simulink model "ChargerSystem"  (R2018a)
settings: Solver=FixedStepDiscrete  StartTime=0.0  StopTime=inf  RelTol=1e-3
libraries: arduinolib x8, simulink x1
settings Model: SimulationMode=external  ExtModeTrigDuration=2  Creator=fabricek  LastModifiedBy=fabricek
settings SolverCC: AutoInsertRateTranBlk=on
settings DataIOCC: SignalLogging=off
settings OptimizationCC: EnhancedBackFolding=on  PassReuseOutputArgsThreshold=0  MaxStackSize=64  OptimizeBlockOrder=speed  DifferentSizesBufferReuse=on  OptimizationCustomize=off
settings DebuggingCC: ParameterTunabilityLossMsg=error
settings HardwareCC: ProdBitPerInt=16  ProdBitPerPointer=16  ProdBitPerSizeT=16  ProdBitPerPtrDiffT=16  ProdLargestAtomicFloat=None  ProdWordSize=8  ProdHWDeviceType=Atmel->AVR  UseEmbeddedCoderFeatures=off  UseSimulinkCoderFeatures=off
settings SFSimCC: MATLABDynamicMemAlloc=off
settings RTWCC: SystemTargetFile=ert.tlc  HardwareBoard=Arduino Uno  TLCOptions=-aInlineSetEventsForThisBaseRateFcn=TLC_FALSE -aSuppressMultiTaskScheduler=TLC_FALSE -aRateBasedStepFcn=1  TemplateMakefile=ert_default_tmf  GenerateReport=on  Toolchain=Arduino AVR  BuildConfiguration=Faster Runs  LaunchReport=on
settings CodeAppCC: ForceParamTrailComments=on  OperatorAnnotations=on
settings ERTTargetCC: ERTCustomFileBanners=off  SupportContinuousTime=on  SupportNonInlinedSFcns=on  RemoveResetFunc=off  SupportVariableSizeSignals=on  ModelStepFunctionPrototypeControlCompliant=off

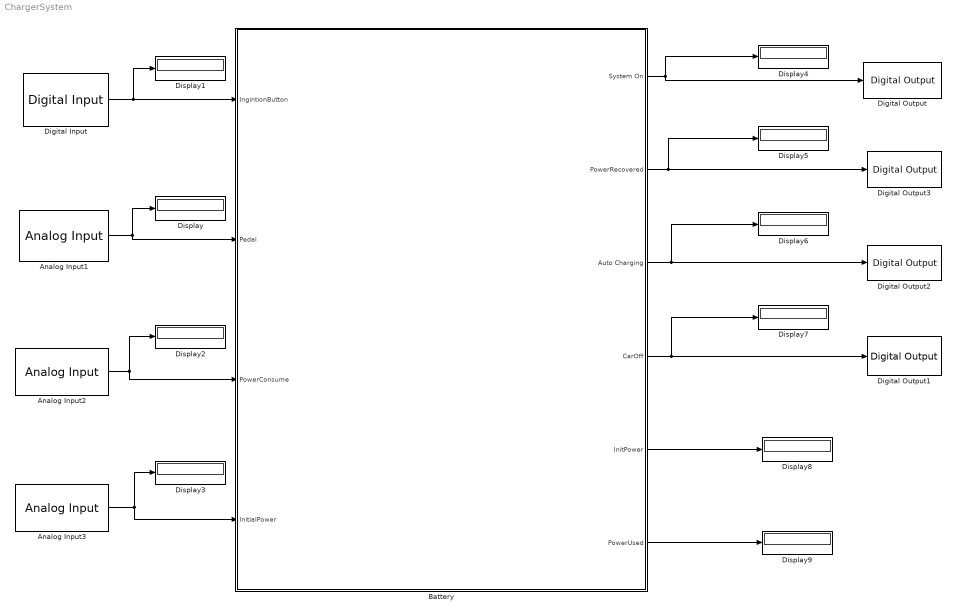
== system ChargerSystem ==
  Analog Input1 : arduinolib/Analog Input  pinNumber=2  ReadResultsOnly=off  ConversionTriggerSource=Software  ExternalTriggerType=uint32(0)  OutputDataType=uint16  EnableConversionCompleteNotify=off  EnableOuputStatus=off  SampleTime=1  blockPlatform=arduino
  Analog Input2 : arduinolib/Analog Input  pinNumber=1  ReadResultsOnly=off  ConversionTriggerSource=Software  ExternalTriggerType=uint32(0)  OutputDataType=uint16  EnableConversionCompleteNotify=off  EnableOuputStatus=off  SampleTime=1  blockPlatform=arduino
  Analog Input3 : arduinolib/Analog Input  pinNumber=0  ReadResultsOnly=off  ConversionTriggerSource=Software  ExternalTriggerType=uint32(0)  OutputDataType=uint16  EnableConversionCompleteNotify=off  EnableOuputStatus=off  SampleTime=1  blockPlatform=arduino
  Battery : Subsystem
  Digital Input : arduinolib/Digital Input  pinNumber=13  sampleTime=0.1  blockPlatform=arduino
      settings: SourceProductName=Simulink Support Package for Arduino Hardware
  Digital Output : arduinolib/Digital Output  pinNumber=9  blockPlatform=arduino
  Digital Output1 : arduinolib/Digital Output  pinNumber=2  blockPlatform=arduino
  Digital Output2 : arduinolib/Digital Output  pinNumber=4  blockPlatform=arduino
  Digital Output3 : arduinolib/Digital Output  pinNumber=7  blockPlatform=arduino
  Display{,1..9} (10 alike) : Display
  wires:
  Battery/6(PowerUsed) -> Display9/1
  Analog Input2/1 -> Battery/3(PowerConsume), Display2/1
  Battery/2(PowerRecovered) -> Display5/1, Digital Output3/1
  Analog Input3/1 -> Battery/4(InitialPower), Display3/1
  Battery/5(InitPower) -> Display8/1
  Battery/1(System On) -> Digital Output/1, Display4/1
  Battery/3(Auto Charging) -> Display6/1, Digital Output2/1
  Battery/4(CarOff) -> Display7/1, Digital Output1/1
  Analog Input1/1 -> Battery/2(Pedal), Display/1
  Digital Input/1 -> Battery/1(IngintionButton), Display1/1

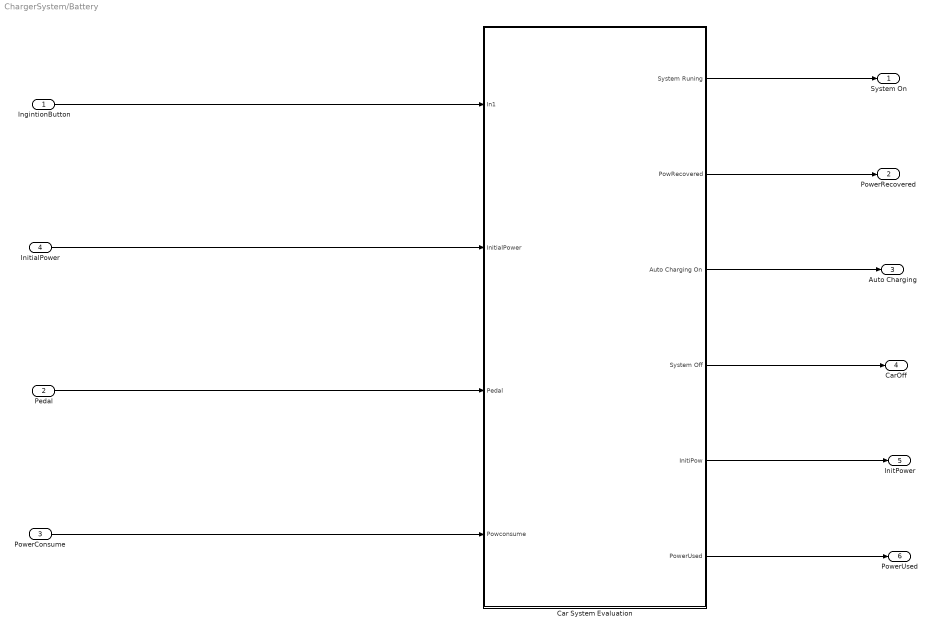
== system ChargerSystem/Battery ==
  IngintionButton : Inport
  Pedal : Inport  Port=2
  PowerConsume : Inport  Port=3
  InitialPower : Inport  Port=4
  Car System Evaluation : Subsystem
  System On : Outport
  PowerRecovered : Outport  Port=2
  Auto Charging : Outport  Port=3
  CarOff : Outport  Port=4
  InitPower : Outport  Port=5
  PowerUsed : Outport  Port=6
  wires:
  IngintionButton/1 -> Car System Evaluation/1(In1)
  Car System Evaluation/4(System Off) -> CarOff/1
  Car System Evaluation/1(System Runing) -> System On/1
  Car System Evaluation/2(PowRecovered) -> PowerRecovered/1
  Car System Evaluation/3(Auto Charging On) -> Auto Charging/1
  Pedal/1 -> Car System Evaluation/3(Pedal)
  PowerConsume/1 -> Car System Evaluation/4(Powconsume)
  InitialPower/1 -> Car System Evaluation/2(InitialPower)
  Car System Evaluation/5(InitiPow) -> InitPower/1
  Car System Evaluation/6(PowerUsed) -> PowerUsed/1

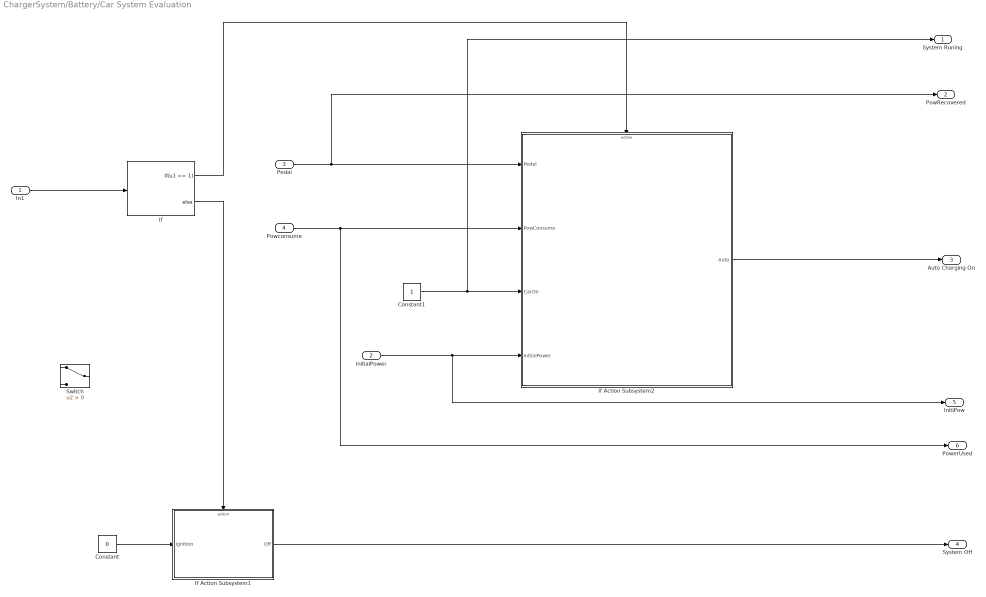
== system ChargerSystem/Battery/Car System Evaluation ==
  In1 : Inport
  InitialPower : Inport  Port=2
  Pedal : Inport  Port=3  LockScale=on
  Powconsume : Inport  Port=4
  Constant : Constant  Value=0
  Constant1 : Constant
  If : If  IfExpression=u1 == 1
  If Action Subsystem1 : Subsystem  TreatAsAtomicUnit=on
  If Action Subsystem2 : Subsystem  TreatAsAtomicUnit=on
  Switch : Switch  Criteria=u2 > Threshold
  System Runing : Outport
  PowRecovered : Outport  Port=2
  Auto Charging On : Outport  Port=3
  System Off : Outport  Port=4
  InitiPow : Outport  Port=5
  PowerUsed : Outport  Port=6
  wires:
  If Action Subsystem1/1(Off) -> System Off/1
  In1/1 -> If/1
  If Action Subsystem2/1(Auto) -> Auto Charging On/1
  If/1 -> If Action Subsystem2/Action
  If/2 -> If Action Subsystem1/Action
  Pedal/1 -> If Action Subsystem2/1(Pedal), PowRecovered/1
  Powconsume/1 -> If Action Subsystem2/2(PowConsume), PowerUsed/1
  InitialPower/1 -> If Action Subsystem2/4(InitialPower), InitiPow/1
  Constant/1 -> If Action Subsystem1/1(Ignition)
  Constant1/1 -> If Action Subsystem2/3(CarOn), System Runing/1

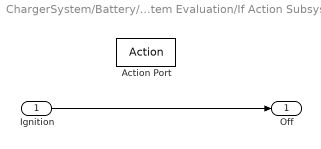
== system ChargerSystem/Battery/Car System Evaluation/If Action Subsystem1 ==
  Ignition : Inport
  Action Port : ActionPort  ActionType=else
  Off : Outport
  wires:
  Ignition/1 -> Off/1

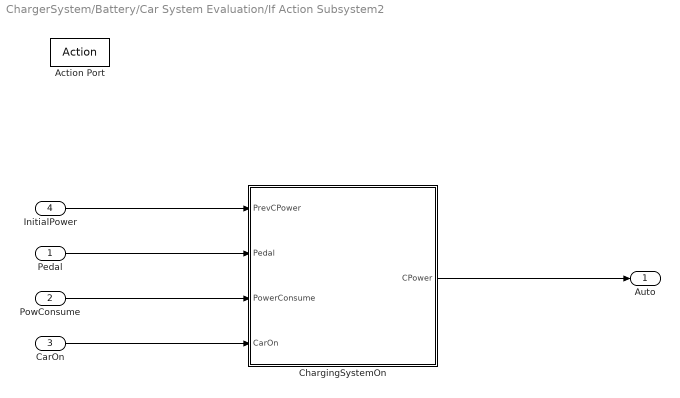
== system ChargerSystem/Battery/Car System Evaluation/If Action Subsystem2 ==
  Pedal : Inport
  PowConsume : Inport  Port=2
  CarOn : Inport  Port=3
  InitialPower : Inport  Port=4
  Action Port : ActionPort  InitializeStates=reset  ActionType=then
  ChargingSystemOn : Subsystem  TreatAsAtomicUnit=on
  Auto : Outport
  wires:
  PowConsume/1 -> ChargingSystemOn/3(PowerConsume)
  ChargingSystemOn/1(CPower) -> Auto/1
  Pedal/1 -> ChargingSystemOn/2(Pedal)
  CarOn/1 -> ChargingSystemOn/4(CarOn)
  InitialPower/1 -> ChargingSystemOn/1("   PrevCPower")

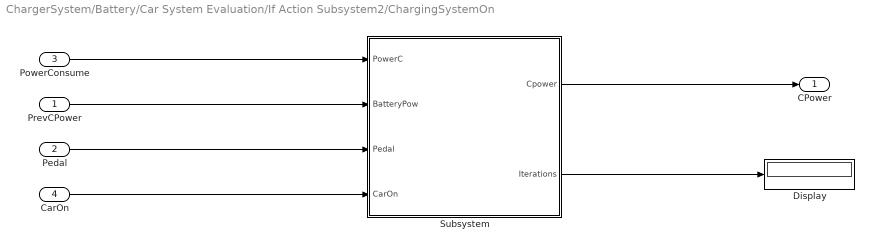
== system ChargerSystem/Battery/Car System Evaluation/If Action Subsystem2/ChargingSystemOn ==
  "   PrevCPower" : Inport
  Pedal : Inport  Port=2
  PowerConsume : Inport  Port=3
  CarOn : Inport  Port=4
  Display : Display
  Subsystem : Subsystem
  CPower : Outport
  wires:
  PowerConsume/1 -> Subsystem/1("   PowerC")
  "   PrevCPower"/1 -> Subsystem/2(BatteryPow)
  Pedal/1 -> Subsystem/3(Pedal)
  Subsystem/1(Cpower) -> CPower/1
  Subsystem/2(Iterations) -> Display/1
  CarOn/1 -> Subsystem/4(CarOn)

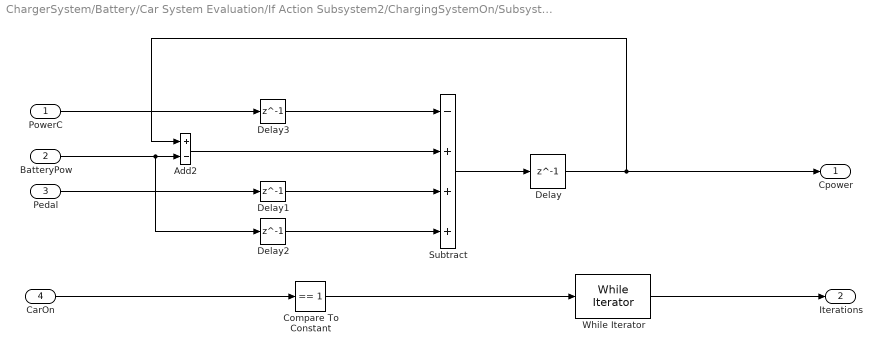
== system ChargerSystem/Battery/Car System Evaluation/If Action Subsystem2/ChargingSystemOn/Subsystem ==
  "   PowerC" : Inport
  BatteryPow : Inport  Port=2
  Pedal : Inport  Port=3
  CarOn : Inport  Port=4
  Add2 : Sum  Inputs=+-
  Compare To Constant : simulink/Logic and Bit Operations/Compare To Constant  relop===  const=1  OutDataTypeStr=boolean
  Delay{,1..3} (4 alike) : Delay  DelayLength=1
  Subtract : Sum  Inputs=-+++
  While Iterator : WhileIterator  MaxIters=500  WhileBlockType=do-while  ShowIterationPort=on
  Cpower : Outport
  Iterations : Outport  Port=2
  wires:
  BatteryPow/1 -> Add2/2, Delay2/1
  Add2/1 -> Subtract/2
  Compare To Constant/1 -> While Iterator/1
  While Iterator/1 -> Iterations/1
  Subtract/1 -> Delay/1
  Delay/1 -> Add2/1, Cpower/1
  Delay2/1 -> Subtract/4
  "   PowerC"/1 -> Delay3/1
  Delay3/1 -> Subtract/1
  CarOn/1 -> Compare To Constant/1
  Pedal/1 -> Delay1/1
  Delay1/1 -> Subtract/3
